simulink model "SCPF_simple"  (R2018b)
settings: Solver=VariableStepAuto  StartTime=0.0  StopTime=100  MaxStep=1e-4  RelTol=1e-16
values from neighbouring files (symbols this model uses):
  seed = 1    [Network_configuration.m]
undefined symbols (not defined in the file or in its folder): advArrivalRate, entity, m, n, release, share1, weightScheme
libraries: simulink x2
settings Model: SimulationMode=accelerator  Creator=Jiaxiao Zheng  LastModifiedBy=Jiaxiao Zheng
settings SolverCC: ZeroCrossAlgorithm=Adaptive

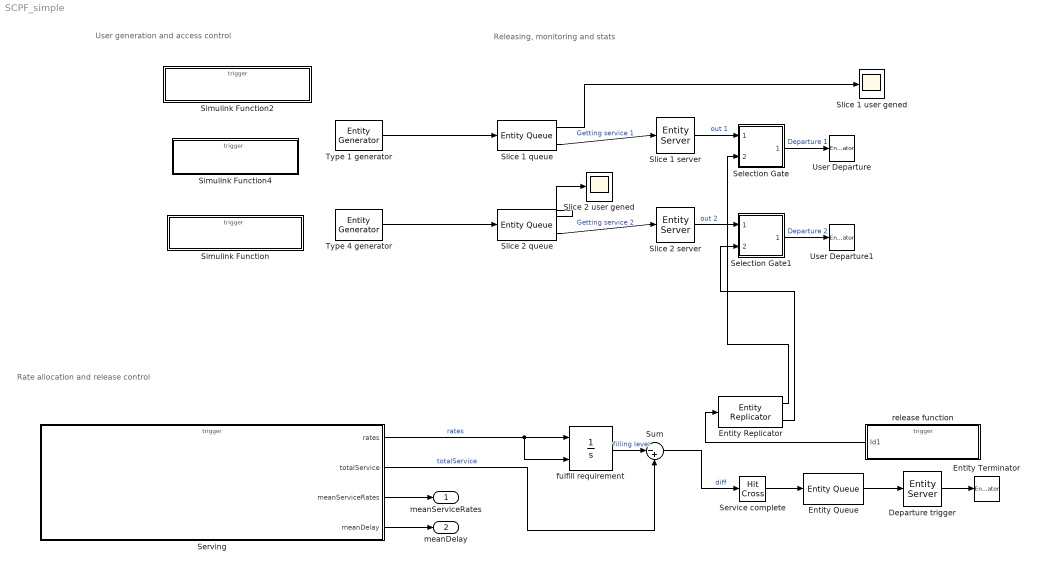
== system SCPF_simple ==
  note: Releasing, monitoring and stats
  note: Rate allocation and release control
  note: User generation and access control
  " Slice 1 server" : EntityServer  InputPortMessageModes=m  OutputPortMessageModes=m  Capacity=50  ServiceTimeValue=0  EntryAction=|
      | assert(size(entity.Id, 1) == 1);
      | assert(size(entity.Id, 2) == 1);
      | assert(entity.Slice == 1);
      | [entity.arrival, entity.socketId] = serving(-1, ...
      |     entity.ServiceTime, 1, entity.Type, 1);
  " Slice 2 server" : EntityServer  InputPortMessageModes=m  OutputPortMessageModes=m  Capacity=50  ServiceTimeValue=0  EntryAction=|
      | assert(size(entity.Id, 1) == 1);
      | assert(size(entity.Id, 2) == 1);
      | assert(entity.Slice == 2);
      | [entity.arrival, entity.socketId] = serving(-1, ...
      |     entity.ServiceTime, 2, entity.Type, 1);
  Departure trigger : EntityServer  InputPortMessageModes=m  OutputPortMessageModes=m  Capacity=100  ServiceTimeValue=0  EntryAction=|  ServiceCompleteAction=release(double(entity.Index));
      | % mark a user as depart
      | % here the entity.Index is the 
      | % id of socket.
      | serving(double(entity.Index), 0, 0, 0, -1);
  Entity Queue : EntityQueue  InputPortMessageModes=m  OutputPortMessageModes=m  Capacity=inf
      settings: OutputPortMap=o5
  Entity Replicator : EntityReplicator  InputPortMessageModes=m  OutputPortMessageModes=m,m
  Entity Terminator : EntityTerminator  InputPortMessageModes=m
  Selection Gate : Subsystem
  Selection Gate1 : Subsystem
  Service complete : HitCross  OutputPortMessageModes=m  HitCrossingDirection=falling  HitCrossingOutputType=Message
  Serving : Subsystem  TreatAsAtomicUnit=on
  Simulink Function : Subsystem  TreatAsAtomicUnit=on
  Simulink Function2 : Subsystem  TreatAsAtomicUnit=on
  Simulink Function4 : Subsystem  TreatAsAtomicUnit=on
  Slice 1 queue : EntityQueue  InputPortMessageModes=m  OutputPortMessageModes=n,m  Capacity=10000  NumberEntitiesDeparted=on
      settings: OutputPortMap=o0,o5
  Slice 1 user gened : Scope
  Slice 2 queue : EntityQueue  InputPortMessageModes=m  OutputPortMessageModes=n,m  Capacity=10000  NumberEntitiesDeparted=on
      settings: OutputPortMap=o0,o5
  Slice 2 user gened : Scope
  Sum : Sum  Inputs=|-+  AccumDataTypeStr=double  OutDataTypeStr=double
  Type 1 generator : EntityGenerator  OutputPortMessageModes=m  TimeSource=MATLAB action  IntergenerationTimeAction=dt = exponentialArrivalTime(1);  GenerateEntityAtSimulationStart=off  GenerateAction=|  AttributeName=ServiceTime|Id|Slice|Type|arrival|departure|socketId  AttributeInitialValue=1|1|1|1|0|0|-1  EntityType=Structured  EntityTypeName=Entity
      | entity.ServiceTime = serviceTime(1);
      | entity.Id = idAllocation();
  Type 4 generator : EntityGenerator  OutputPortMessageModes=m  TimeSource=MATLAB action  IntergenerationTimeAction=dt = exponentialArrivalTime(2);  GenerateEntityAtSimulationStart=off  GenerateAction=|  AttributeName=ServiceTime|Id|Slice|Type|arrival|departure|socketId  AttributeInitialValue=1|1|2|2|1|1|-1  EntityType=Structured  EntityTypeName=Entity
      | entity.ServiceTime = serviceTime(2);
      | entity.Id = idAllocation();
  User Departure : EntityTerminator  InputPortMessageModes=m
  User Departure1 : EntityTerminator  InputPortMessageModes=m
  fulfill requirement : Integrator  ExternalReset=falling
  release function : Subsystem  TreatAsAtomicUnit=on
  meanServiceRates : Outport
  meanDelay : Outport  Port=2
  wires:
  Slice 1 queue/2 -> " Slice 1 server"/1  "Getting service 1"
  " Slice 1 server"/1 -> Selection Gate/1(User)  "out 1"
  Selection Gate/1(Out1) -> User Departure/1  "Departure 1"
  Serving/1(rates) -> fulfill requirement/1, fulfill requirement/2  "rates"
  Serving/2(totalService) -> Sum/2  "totalService"
  fulfill requirement/1 -> Sum/1  "filling level"
  Sum/1 -> Service complete/1  "diff"
  Service complete/1 -> Entity Queue/1
  Entity Queue/1 -> Departure trigger/1
  Departure trigger/1 -> Entity Terminator/1
  Slice 2 queue/2 -> " Slice 2 server"/1  "Getting service 2"
  " Slice 2 server"/1 -> Selection Gate1/1(User)  "out 2"
  Selection Gate1/1(Out1) -> User Departure1/1  "Departure 2"
  release function/1(Id1) -> Entity Replicator/1
  Entity Replicator/1 -> Selection Gate/2(UserId)
  Entity Replicator/2 -> Selection Gate1/2(UserId)
  Slice 1 queue/1 -> Slice 1 user gened/1
  Slice 2 queue/1 -> Slice 2 user gened/1
  Serving/3(meanServiceRates) -> meanServiceRates/1
  Serving/4(meanDelay) -> meanDelay/1
  Type 1 generator/1 -> Slice 1 queue/1
  Type 4 generator/1 -> Slice 2 queue/1

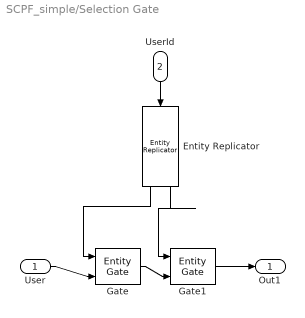
== system SCPF_simple/Selection Gate ==
  User : Inport
  UserId : Inport  Port=2
  Entity Replicator : EntityReplicator  InputPortMessageModes=m  OutputPortMessageModes=m,m
  Gate : EntityGate  InputPortMessageModes=m,m  OutputPortMessageModes=m  OperatingMode=Selection gate  MatchingAttributeName=socketId
  Gate1 : EntityGate  InputPortMessageModes=m,m  OutputPortMessageModes=m  OperatingMode=Release gate  MatchingAttributeName=Id
  Out1 : Outport
  wires:
  Gate/1 -> Gate1/2
  Entity Replicator/1 -> Gate/1
  Entity Replicator/2 -> Gate1/1
  Gate1/1 -> Out1/1
  User/1 -> Gate/2
  UserId/1 -> Entity Replicator/1

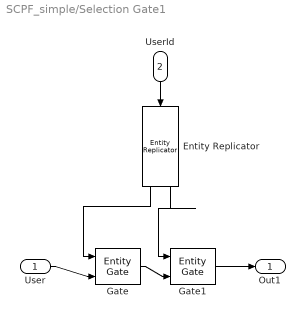
== system SCPF_simple/Selection Gate1 ==
  User : Inport
  UserId : Inport  Port=2
  Entity Replicator : EntityReplicator  InputPortMessageModes=m  OutputPortMessageModes=m,m
  Gate : EntityGate  InputPortMessageModes=m,m  OutputPortMessageModes=m  OperatingMode=Selection gate  MatchingAttributeName=socketId
  Gate1 : EntityGate  InputPortMessageModes=m,m  OutputPortMessageModes=m  OperatingMode=Release gate  MatchingAttributeName=Id
  Out1 : Outport
  wires:
  Gate/1 -> Gate1/2
  Entity Replicator/1 -> Gate/1
  Entity Replicator/2 -> Gate1/1
  Gate1/1 -> Out1/1
  User/1 -> Gate/2
  UserId/1 -> Entity Replicator/1

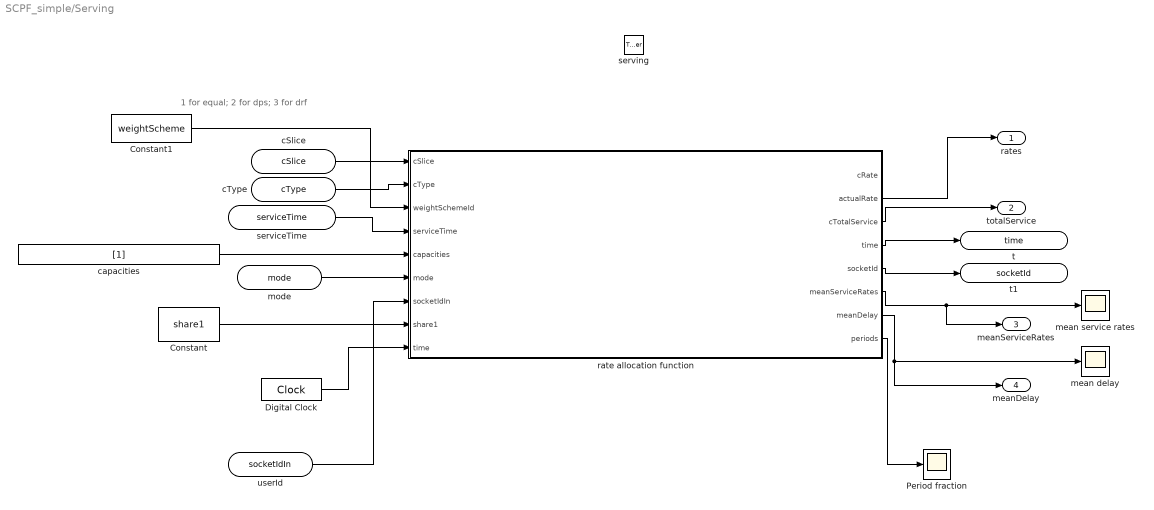
== system SCPF_simple/Serving ==
  note: 1 for equal; 2 for dps; 3 for drf
  serving : TriggerPort  TriggerType=function-call  IsSimulinkFunction=on  FunctionName=serving  VariantControl=(inherit)
  Constant : Constant  Value=share1
  Constant1 : Constant  Value=weightScheme
  Digital Clock : DigitalClock  SampleTime=-1
  Period fraction : Scope
  capacities : Constant  Value=[1]
  mean delay : Scope
  mean service rates : Scope
  rate allocation function : MATLAB Function  TreatAsAtomicUnit=on
  userId : ArgIn  DisableCoverage=on  ArgumentName=socketIdIn
  serviceTime : ArgIn  DisableCoverage=on  Port=2  ArgumentName=serviceTime
  cSlice : ArgIn  DisableCoverage=on  Port=3  ArgumentName=cSlice
  cType : ArgIn  DisableCoverage=on  Port=4  ArgumentName=cType
  mode : ArgIn  DisableCoverage=on  Port=5  ArgumentName=mode
  t : ArgOut  DisableCoverage=on  ArgumentName=time
  t1 : ArgOut  DisableCoverage=on  Port=2  ArgumentName=socketId
  rates : Outport  SourceOfInitialOutputValue=Input signal
  totalService : Outport  Port=2  OutDataTypeStr=double
  meanServiceRates : Outport  Port=3
  meanDelay : Outport  Port=4
  wires:
  serviceTime/1 -> rate allocation function/4(serviceTime)
  capacities/1 -> rate allocation function/5(capacities)
  cSlice/1 -> rate allocation function/1(cSlice)
  cType/1 -> rate allocation function/2(cType)
  mode/1 -> rate allocation function/6(mode)
  rate allocation function/3(cTotalService) -> totalService/1
  Constant/1 -> rate allocation function/8(share1)
  rate allocation function/4(time) -> t/1
  Digital Clock/1 -> rate allocation function/9("time ")
  rate allocation function/5(socketId) -> t1/1
  userId/1 -> rate allocation function/7(socketIdIn)
  rate allocation function/6(meanServiceRates) -> meanServiceRates/1, mean service rates/1
  Constant1/1 -> rate allocation function/3(weightSchemeId)
  rate allocation function/7(meanDelay) -> meanDelay/1, mean delay/1
  rate allocation function/8(periods) -> Period fraction/1
  rate allocation function/2(actualRate) -> rates/1

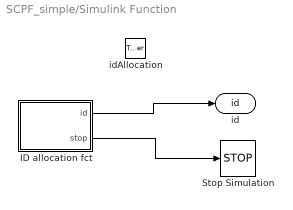
== system SCPF_simple/Simulink Function ==
  idAllocation : TriggerPort  TriggerType=function-call  IsSimulinkFunction=on  FunctionName=idAllocation  VariantControl=(inherit)
  " ID allocation fct" : MATLAB Function  TreatAsAtomicUnit=on
  Stop Simulation : Stop
  id : ArgOut  DisableCoverage=on  ArgumentName=id
  wires:
  " ID allocation fct"/1(id) -> id/1
  " ID allocation fct"/2(stop) -> Stop Simulation/1

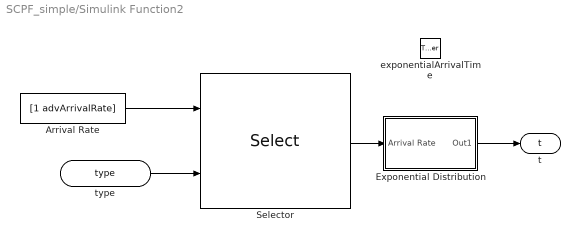
== system SCPF_simple/Simulink Function2 ==
  exponentialArrivalTime : TriggerPort  TriggerType=function-call  IsSimulinkFunction=on  FunctionName=exponentialArrivalTime  VariantControl=Variant
  Arrival Rate : Constant  Value=[1 advArrivalRate]  SampleTime=-1
  Exponential Distribution : Subsystem
  Selector : Selector  IndexOptions=Index vector (port)  Indices=[1 3]  OutputSizes=1
  type : ArgIn  DisableCoverage=on  ArgumentName=type
  t : ArgOut  DisableCoverage=on  ArgumentName=t
  wires:
  Exponential Distribution/1(Out1) -> t/1
  Arrival Rate/1 -> Selector/1
  Selector/1 -> Exponential Distribution/1(Arrival Rate)
  type/1 -> Selector/2

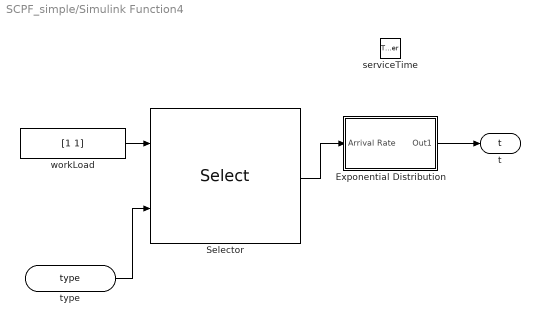
== system SCPF_simple/Simulink Function4 ==
  serviceTime : TriggerPort  TriggerType=function-call  IsSimulinkFunction=on  FunctionName=serviceTime  VariantControl=Variant
  Exponential Distribution : Subsystem
  Selector : Selector  IndexOptions=Index vector (port)  Indices=[1 3]  OutputSizes=1
  workLoad : Constant  Value=[1 1]  SampleTime=-1
  type : ArgIn  DisableCoverage=on  ArgumentName=type
  t : ArgOut  DisableCoverage=on  ArgumentName=t
  wires:
  Exponential Distribution/1(Out1) -> t/1
  type/1 -> Selector/2
  workLoad/1 -> Selector/1
  Selector/1 -> Exponential Distribution/1(Arrival Rate)

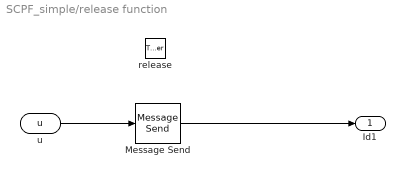
== system SCPF_simple/release function ==
  release : TriggerPort  TriggerType=function-call  IsSimulinkFunction=on  FunctionName=release  VariantControl=(inherit)
  Message Send : MessageSend  OutputPortMessageModes=m
      settings: InputPortMap=u1
  u : ArgIn  DisableCoverage=on  ArgumentName=u
  Id1 : Outport
  wires:
  u/1 -> Message Send/1
  Message Send/1 -> Id1/1

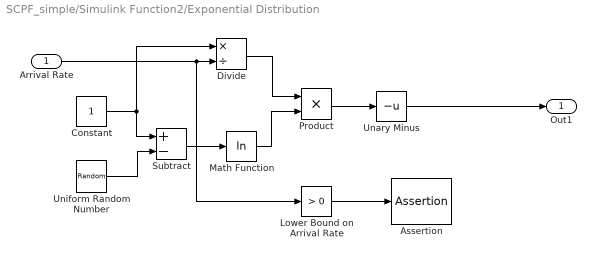
== system SCPF_simple/Simulink Function2/Exponential Distribution ==
  Arrival Rate : Inport
  Assertion : Assertion
  Constant : Constant
  Divide : Product  Inputs=*/
  Lower Bound on Arrival Rate : simulink/Logic and Bit Operations/Compare To Constant  relop=>  const=0  OutDataTypeStr=uint8  ZeroCross=off
  Math Function : Math  Operator=log  SaturateOnIntegerOverflow=on
  Product : Product  RndMeth=Zero
  Subtract : Sum  Inputs=+-
  Unary Minus : UnaryMinus
  Uniform Random Number : UniformRandomNumber  Minimum=0  Seed=seed
  Out1 : Outport
  wires:
  Subtract/1 -> Math Function/1
  Lower Bound on Arrival Rate/1 -> Assertion/1
  Uniform Random Number/1 -> Subtract/2
  Constant/1 -> Subtract/1, Divide/1
  Divide/1 -> Product/1
  Math Function/1 -> Product/2
  Product/1 -> Unary Minus/1
  Unary Minus/1 -> Out1/1
  Arrival Rate/1 -> Lower Bound on Arrival Rate/1, Divide/2

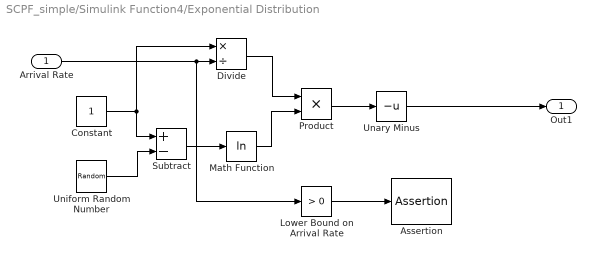
== system SCPF_simple/Simulink Function4/Exponential Distribution ==
  Arrival Rate : Inport
  Assertion : Assertion
  Constant : Constant
  Divide : Product  Inputs=*/
  Lower Bound on Arrival Rate : simulink/Logic and Bit Operations/Compare To Constant  relop=>  const=0  OutDataTypeStr=uint8  ZeroCross=off
  Math Function : Math  Operator=log  SaturateOnIntegerOverflow=on
  Product : Product  RndMeth=Zero
  Subtract : Sum  Inputs=+-
  Unary Minus : UnaryMinus
  Uniform Random Number : UniformRandomNumber  Minimum=0  Seed=12345
  Out1 : Outport
  wires:
  Subtract/1 -> Math Function/1
  Lower Bound on Arrival Rate/1 -> Assertion/1
  Uniform Random Number/1 -> Subtract/2
  Constant/1 -> Subtract/1, Divide/1
  Divide/1 -> Product/1
  Math Function/1 -> Product/2
  Product/1 -> Unary Minus/1
  Unary Minus/1 -> Out1/1
  Arrival Rate/1 -> Lower Bound on Arrival Rate/1, Divide/2

== matlab function SCPF_simple/Serving/rate allocation function ==
  data: cSlice input; cType input; weightSchemeId input; cRate output double size=[1, 100]; actualRate output double size=[1, 100]; serviceTime input; capacities input; mode input; socketIdIn input; cTotalService output double size=[1, 100]; share1 input; time input; time output; socketId output; meanServiceRates output; meanDelay output; periods output
function [cRate, actualRate, cTotalService, time, socketId, meanServiceRates, ...
    meanDelay, periods] = rateAllocation(cSlice, cType, weightSchemeId, ...
    serviceTime, capacities, mode, socketIdIn, share1, time)
% Parameters:
% userId: current incoming user's id, scalar
% serviceTime: the service requirement of the incoming user, R x 1 vector.
% capacities: capacities of the resources, R x 1 vector
% share: share for each slice, 1 x V
% mode: 1 = arrival, -1 = departure 
% socketIdIn: if departure, which socket is being released.

% Persistent vars:
% userActive: vector of 1 x nSocket, userActive(s) = 1 iff socket s is
% currently working
% userDemands: vector of R x nSocket, userDemands(:, s) is the demand
% vector of the user currently at socket s
% userRates: vector of 1 x nSocket, userRates(s) = current service rate of
% socket s
% userServiceTime: 1 x nSocket, userServiceTime(s) = current service
% requirement of user at socket s
% userSlice: 1 x nSocket, userSlice(s) = the idx of slice of user at socket
% s
% userWeights: 1 x nSocket, user weight allocation across sockets
% R: nResource
% nCumulatedUsers: 1 x V, number of users departed up to now
% nMeanServiceRate: 1 x V, current mean service rate of each slice
% nMeanDelay: 1 x V, current mean delay of each slice
% userArrivalTime: 1 x nSocket, the arrival time of user currently at
% socket s.
% periodDistribution: 1 x 3, (only 1 busy, only 2 busy, both 1and2 busy)
% prevTime: last timestamp, in order to compute duration.
persistent userActive userDemands userRates userServiceTime userSlice ...
    userWeights R nCumulatedUsers nMeanServiceRate nMeanDelay ...
    userArrivalTime periodDistribution prevTime;

% predefined demanding vector for each type,
typeDemands = [1;1];

share = [share1 1 - share1]';
windowSize = 100;

% function to solve maxmin problem
%---------------------------Begin nested function--------------------------
    function [ rates ] = maxminsolve(mmweights, mmcapacities, demands)
    % Solve the maxmin rate allocation problem under the resource constraint.
    % 
    % max  min_i r_i/w_i
    % s.t. sum_i d(i, j) r_i <= c_j for each j
    %
    % Assuming everyone has nonzero weights and demands.
    % --------------------------------
    % Parameters:
    % --------------------------------
    % - weights: array of user weights, nUsers x 1 matrix
    % - capacities: array of resources capacities, R x 1 matrix
    % - demands: resource demands per user, R x nUsers matrix
    % --------------------------------
    % Ret:
    % --------------------------------
    % - rate: rate allocation to each user, 1 x nUsers matrix

    N = size(mmweights, 2); % number of users.
    if N == 0
        rates = 0;
        return
    end

    rates = zeros(1, N);
    remainingCap = mmcapacities;
    bottlenecked = zeros(1, N); % none of the users are bottlenecked
    bottleneckedResource = zeros(1, R);

    while(max(remainingCap) > 1e-7 && min(bottlenecked) == 0 && ...
            min(bottleneckedResource) == 0)
        activeRemainingCap = remainingCap;
        activeRemainingCap(bottleneckedResource > 0) = inf;
        weightedDemands = zeros(R, 1);
        for i = 1:N
            for r = 1:R
                % if any of the resource it needs is bottlenecked,
                % this user is also BNed
                if (bottleneckedResource(r) > 0 && demands(r, i) > 0)
                    bottlenecked(i) = 1;
                end
            end
            if (bottlenecked(i) > 0)
                continue;
            end
            for r = 1:R
                weightedDemands(r) = weightedDemands(r) + mmweights(i) ...
                    * demands(r, i);
            end
        end
        [increment, minidx] = min(activeRemainingCap ./ weightedDemands);
        if(increment == inf) % to deal with the case demand orthogonal to 
                             % remaining capacity
            break
        end
        bottleneckedResource(minidx) = 1;
        for i = 1:N
            if(bottlenecked(i) > 0)
                continue;
            end
            rates(i) = rates(i) + increment * mmweights(i);
            % all the users have demand in minidx are bned
            if(demands(minidx, i) > 0)
                bottlenecked(i) = 1;
            end
        end

        for r = 1:R
            if(remainingCap == 0)
                continue;
            end
            remainingCap(r) = remainingCap(r) - weightedDemands(r) * ...
                increment;
            if(abs(remainingCap(r)) < 1e-10)
                remainingCap(r) = 0;
                bottleneckedResource(r) = 1; 
                % needed if two resources get BNed at the same time.
            end
        end      
    end
    end
%---------------------------End nested function----------------------------

% wrapper function avoid zero weights
%---------------------------Begin nested function--------------------------
    function [ rate ] = maxmin(weights, wrapper_capacities, demands)
    % Solve the maxmin rate allocation problem under the resource constraint.
    % Cache is used to improve the simulation speed.
    % --------------------------------
    % Parameters:
    % --------------------------------
    % - userTypes : array of user types, 1 x nUsers matrix
    % - weights: array of user weights, nUsers x 1 matrix
    % - capacities: array of resources capacities, 1 x R matrix
    % - demands: resource demands per user, R x nUsers matrix
    % - cache: a map to store existing results
    % --------------------------------
    % Ret:
    % --------------------------------
    % - rate: rate allocation to each user, 1 x nUsers matrix
    % - lambda: redundant, keep for backward comaptibility.
    % First need to filter out the zeroes in the input
    if max(weights) == 0
        rate = zeros(windowSize, 1);
        return
    end
    nonZeroIdx = find(weights);

    filteredWeights = weights(nonZeroIdx);
    filteredDemands = demands(:, nonZeroIdx);    
    filteredRate = maxminsolve(filteredWeights, ...
        wrapper_capacities, filteredDemands);
    assert(all(filteredRate >= 0));
    % change back
    rate = zeros(size(weights))';
    rate(nonZeroIdx) = filteredRate;
    end
%---------------------------End nested function----------------------------

% function for user weight allocation
%---------------------------Begin nested function--------------------------
    function user_weights = getweightallocation( user_active, ...
            user_demands, shares, weightStrata, capacity, user_slice )
        numSlice = 2;
    % Function that returns user level weight allocation.
    % --------------------------------
    % Parameters:
    % --------------------------------
    % userActive: flag vector marking active users, userActive(i) = 1 if user i
    % is active. 1 x nUser
    % userDemands: resource demand vector of users, R x nUser
    % shares: share allocation among slices, 1 x V
    % weightStrata: string of weighting scheme
    % capacities: capacity of each resource, B x 1
    % user_slice: vector marking which slice each user belongs to, 1 x nUser.
    % --------------------------------
    % Ret:
    % --------------------------------
    % userWeights: weight of each user, 1 x nUser

    % weight allocation corresponds to discrimnatory processor sharing, 
    % slices are not protected against each other
    user_weights = user_active;
    if(strcmp(weightStrata, 'dps'))
        user_weights = user_active;
        for w_id = 1 : windowSize
            if(user_active(w_id) == 1)
                user_weights(w_id) = user_weights(w_id) ...
                    * shares(user_slice(w_id));
            end
        end
    end

    if(strcmp(weightStrata, 'equal'))
        user_weights = user_active;
        w_slice_cnt = zeros(numSlice, 1);
        if(max(user_active) == 0)
            return
        end
        for w_id = 1 : windowSize
            if(user_active(w_id) == 1)
                w_slice_cnt(user_slice(w_id)) = ...
                    w_slice_cnt(user_slice(w_id)) + 1;
            end
        end
        ww_per_slice = shares ./ w_slice_cnt;
        for w_id = 1 : windowSize
            if(user_active(w_id) == 1)
                user_weights(w_id) = ww_per_slice(user_slice(w_id));
            end
        end
    end

    if(strcmp(weightStrata, 'drf'))
        user_weights = user_active;
        
        slice_inverse_ds = zeros(numSlice, 1);
        for w_id = 1 : windowSize
            if(user_active(w_id) == 1)
                dominantSharesVec = user_demands(:, w_id) ./ capacity;
                dominantShare = max(dominantSharesVec);
                slice_inverse_ds(user_slice(w_id)) = ...
                    slice_inverse_ds(user_slice(w_id)) + 1 / dominantShare;
            end
        end
        for w_id = 1 : windowSize
            if(user_active(w_id) == 1)
                dominantSharesVec = user_demands(:, w_id) ./ capacity;
                dominantShare = max(dominantSharesVec);
                user_weights(w_id) = shares(user_slice(w_id)) * (1 ...
                    / dominantShare) / slice_inverse_ds(user_slice(w_id));
            end
        end
    end
    end
%---------------------------End nested function----------------------------

% init
R = size(capacities, 1);

if isempty(userDemands)
    % initialize vectors, if extension needed, double size.
    userDemands = zeros(R, windowSize);
    userActive = zeros(1, windowSize);
    userRates = zeros(1, windowSize);
    userSlice = zeros(1, windowSize);
    userWeights = zeros(1, windowSize);
    userServiceTime = zeros(1, windowSize);
    nCumulatedUsers = zeros(1, 2);
    nMeanServiceRate = zeros(1, 2);
    nMeanDelay = zeros(1, 2);
    userArrivalTime = zeros(1, windowSize);
    periodDistribution = zeros(1, 3);
    prevTime = 0;
end
tsocketId = 0;
weightScheme = 'equal';
switch weightSchemeId
    case 1
        weightScheme = 'equal';
    case 2
        weightScheme = 'dps';
    case 3
        weightScheme = 'drf';
end
switch mode
    case 0 % just mark time
        
    case 1 % arrival
        % need to find the first available socket to plug in
        availableSkt = find(userActive == 0);
        assert(size(availableSkt, 2) > 0);
        firstAvailable = availableSkt(1);
        tsocketId = firstAvailable;
        userDemands(:, tsocketId) = typeDemands(cType, :)';
        userServiceTime(tsocketId) = serviceTime;
        userActive(tsocketId) = 1;
        userSlice(tsocketId) = cSlice;
        userArrivalTime(tsocketId) = time;
        % determine weights
        userWeights = getweightallocation(userActive, userDemands, ...
            share, weightScheme, capacities, userSlice);
        %rate allocation
        userRates = maxmin(userWeights, capacities, userDemands)';
    case -1 % departure
        tsocketId = socketIdIn;
        % update cumulative duration
        nSlice1 = sum(userSlice == 1);
        nSlice2 = sum(userSlice == 2);
        if (nSlice1 > 0 && nSlice2 == 0)
            periodDistribution(1) = periodDistribution(1) + time ...
                - prevTime;
        elseif (nSlice1 == 0 && nSlice2 > 0)
            periodDistribution(2) = periodDistribution(2) + time ...
                - prevTime;
        elseif (nSlice1 > 0 && nSlice2 > 0)
            periodDistribution(3) = periodDistribution(3) + time ...
                - prevTime;
        end
        % update mean service rate
        nCumulatedUsers(userSlice(tsocketId)) = ...
            nCumulatedUsers(userSlice(tsocketId)) + 1;
        nMeanDelay(userSlice(tsocketId)) = ...
            ((nCumulatedUsers(userSlice(tsocketId)) - 1) ...
            * nMeanDelay(userSlice(tsocketId)) + (time ...
            - userArrivalTime(tsocketId))) / ...
            nCumulatedUsers(userSlice(tsocketId));
        % In elastic setting, mean service rate is captured by the expected
        % service rate seen by a typical user, thus equal to the mean of
        % mean service rate across times.
        
        % Current mean rate for the slice
        sliceRates = [];
        cSlice = userSlice(tsocketId);
        for socket = 1:windowSize
            if(userActive(socket) == 1 && userSlice(socket) == cSlice)
                sliceRates = [sliceRates userRates(socket)];
            end
        end
        nMeanServiceRate(userSlice(tsocketId)) = ...
            ((nCumulatedUsers(cSlice) - 1) * nMeanServiceRate(cSlice) ...
            + mean(sliceRates)) / nCumulatedUsers(cSlice);
        userDemands(:, tsocketId) = zeros(R, 1);
        userActive(tsocketId) = 0;
        userSlice(tsocketId) = 0;
        userServiceTime(tsocketId) = -1;
        userArrivalTime(tsocketId) = 0;
        userWeights = getweightallocation(userActive, userDemands, share,...
            weightScheme, capacities, userSlice);
        userRates = maxmin(userWeights, capacities, userDemands)';
end
if (mode == 1 || mode == -1) 
    socketId = tsocketId;
else
    socketId = -1;
end
periods = periodDistribution / time;
prevTime = time;
meanServiceRates = nMeanServiceRate(1:2);
meanDelay = nMeanDelay(1:2);
cRate = userRates(1:100);
actualRate = ones(size(cRate)) .* (cRate > 0); % For inelasticity.
cTotalService = userServiceTime(1:100);
cTotalService = cTotalService(1:100);
end

== matlab function SCPF_simple/Simulink Function/ ID allocation fct ==
  data: id output; stop output
function [id, stop] = fcn
persistent userCnt;
if isempty(userCnt)
    userCnt = 0;
end
userCnt = userCnt + 1;
id = userCnt;
%stop = (id >= 1000);
stop = 0;
